simulink model "formationFlight"  (R2024b)
settings: Solver=ode4  StartTime=0.0  StopTime=30  FixedStep=1e-3  RelTol=1e-3
undefined symbols (not defined in the file or in its folder): MDL
settings Model: Creator=Ismail  LastModifiedBy=Ismail

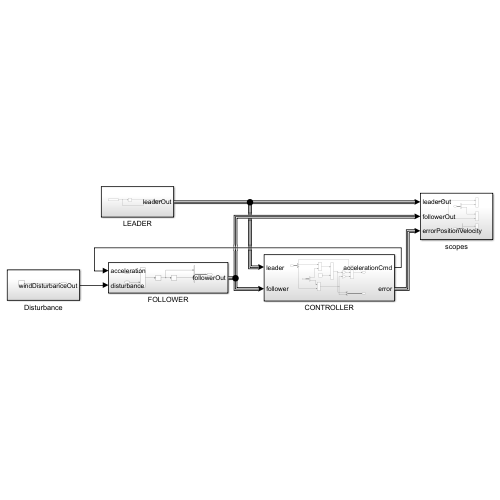
[thumbnail: Simulink's stored preview of the top-level diagram]
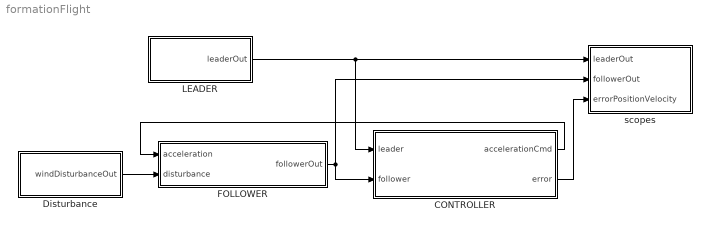
== system formationFlight ==
  CONTROLLER : Subsystem
  Disturbance : Subsystem
  FOLLOWER : Subsystem
  LEADER : Subsystem
  scopes : Subsystem
  wires:
  Disturbance/1(windDisturbanceOut) -> FOLLOWER/2(disturbance)
  LEADER/1(leaderOut) -> scopes/1(leaderOut), CONTROLLER/1(leader)
  FOLLOWER/1(followerOut) -> scopes/2(followerOut), CONTROLLER/2(follower)
  CONTROLLER/1(accelerationCmd) -> FOLLOWER/1(acceleration)
  CONTROLLER/2(error) -> scopes/3(errorPositionVelocity)

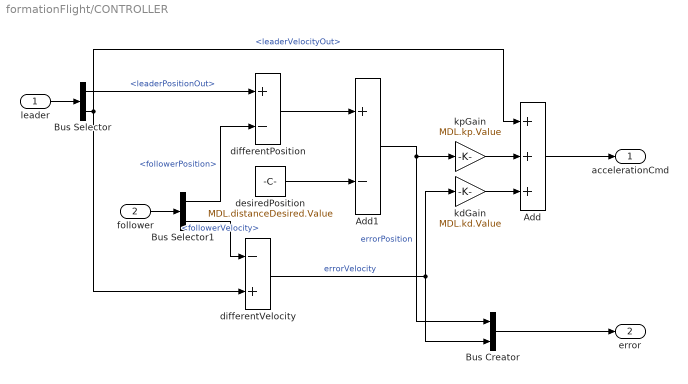
== system formationFlight/CONTROLLER ==
  leader : Inport
  follower : Inport  Port=2
  Add : Sum  Inputs=+++
  Add1 : Sum  Inputs=+-
  Bus Creator : BusCreator  Inputs=2
  Bus Selector : BusSelector  OutputSignals=leaderPositionOut,leaderVelocityOut
  Bus Selector1 : BusSelector  OutputSignals=followerPosition,followerVelocity
  desiredPosition : Constant  Value=MDL.distanceDesired.Value
  differentPosition : Sum  Inputs=+-
  differentVelocity : Sum  Inputs=-+
  kdGain : Gain  Gain=MDL.kd.Value
  kpGain : Gain  Gain=MDL.kp.Value
  accelerationCmd : Outport
  error : Outport  Port=2
  wires:
  differentPosition/1 -> Add1/1
  desiredPosition/1 -> Add1/2
  Add1/1 -> Bus Creator/1, kpGain/1  "errorPosition"
  differentVelocity/1 -> kdGain/1, Bus Creator/2  "errorVelocity"
  kpGain/1 -> Add/2
  kdGain/1 -> Add/3
  Add/1 -> accelerationCmd/1
  follower/1 -> Bus Selector1/1
  leader/1 -> Bus Selector/1
  Bus Selector/1 -> differentPosition/1  "<leaderPositionOut>"
  Bus Selector/2 -> differentVelocity/2, Add/1  "<leaderVelocityOut>"
  Bus Selector1/1 -> differentPosition/2  "<followerPosition>"
  Bus Selector1/2 -> differentVelocity/1  "<followerVelocity>"
  Bus Creator/1 -> error/1

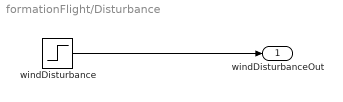
== system formationFlight/Disturbance ==
  windDisturbance : Step  Time=MDL.disturbanceTime.Value  After=-2  SampleTime=0
  windDisturbanceOut : Outport
  wires:
  windDisturbance/1 -> windDisturbanceOut/1

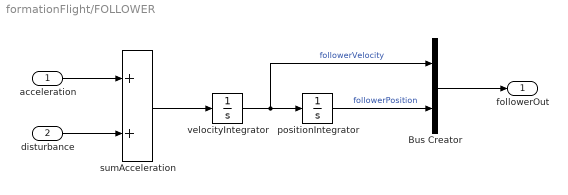
== system formationFlight/FOLLOWER ==
  acceleration : Inport
  disturbance : Inport  Port=2
  Bus Creator : BusCreator  Inputs=2
  positionIntegrator : Integrator  InitialCondition=MDL.followerPositionInit.Value
  sumAcceleration : Sum
  velocityIntegrator : Integrator  InitialCondition=MDL.followerVelocityInit.Value
  followerOut : Outport
  wires:
  acceleration/1 -> sumAcceleration/1
  disturbance/1 -> sumAcceleration/2
  sumAcceleration/1 -> velocityIntegrator/1
  velocityIntegrator/1 -> Bus Creator/1, positionIntegrator/1  "followerVelocity"
  positionIntegrator/1 -> Bus Creator/2  "followerPosition"
  Bus Creator/1 -> followerOut/1

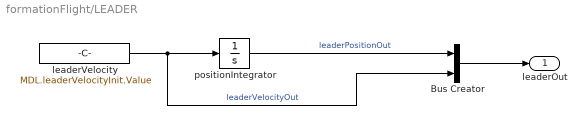
== system formationFlight/LEADER ==
  Bus Creator : BusCreator  Inputs=2
  leaderVelocity : Constant  Value=MDL.leaderVelocityInit.Value
  positionIntegrator : Integrator  InitialCondition=MDL.leaderPositionInit.Value
  leaderOut : Outport
  wires:
  positionIntegrator/1 -> Bus Creator/1  "leaderPositionOut"
  leaderVelocity/1 -> Bus Creator/2, positionIntegrator/1  "leaderVelocityOut"
  Bus Creator/1 -> leaderOut/1

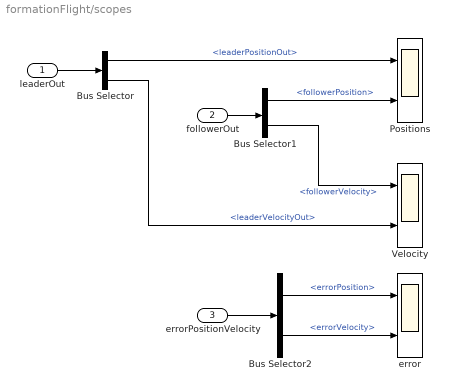
== system formationFlight/scopes ==
  leaderOut : Inport
  followerOut : Inport  Port=2
  errorPositionVelocity : Inport  Port=3
  Bus Selector : BusSelector  OutputSignals=leaderPositionOut,leaderVelocityOut
  Bus Selector1 : BusSelector  OutputSignals=followerPosition,followerVelocity
  Bus Selector2 : BusSelector  OutputSignals=errorPosition,errorVelocity
  Positions : Scope  NumInputPorts=2
  Velocity : Scope  NumInputPorts=2
  error : Scope  NumInputPorts=2
  wires:
  leaderOut/1 -> Bus Selector/1
  Bus Selector/1 -> Positions/1  "<leaderPositionOut>"
  Bus Selector/2 -> Velocity/2  "<leaderVelocityOut>"
  followerOut/1 -> Bus Selector1/1
  Bus Selector1/1 -> Positions/2  "<followerPosition>"
  Bus Selector1/2 -> Velocity/1  "<followerVelocity>"
  errorPositionVelocity/1 -> Bus Selector2/1
  Bus Selector2/1 -> error/1  "<errorPosition>"
  Bus Selector2/2 -> error/2  "<errorVelocity>"
